simulink model "System_1"  (R2017a)
settings: Solver=VariableStepAuto  StartTime=0.0  StopTime=100  MaxStep=0.01  RelTol=1e-3
values from neighbouring files (symbols this model uses):
  ku = 8.4678    [System1.m]
  r_t = b    (= 5)    [System1.m]
libraries: cstblocks x1
settings Model: Creator=dplascen  LastModifiedBy=dplascen
settings HardwareCC: ProdBitPerPointer=32  ProdBitPerSizeT=32  ProdBitPerPtrDiffT=32  ProdWordSize=32  ProdHWDeviceType=Intel->x86-32 (Windows32)

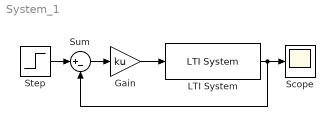
== system System_1 ==
  Gain : Gain  Gain=ku
  LTI System : cstblocks/LTI System  sys=G  IC=[]
  Scope : Scope
  Step : Step  Time=0  After=r_t  SampleTime=0
  Sum : Sum  Inputs=|+-
  wires:
  LTI System/1 -> Sum/2, Scope/1
  Gain/1 -> LTI System/1
  Step/1 -> Sum/1
  Sum/1 -> Gain/1
